simulink model "CheckMate_clipboard"  (R2013a)
settings: Solver=ode23t  StartTime=0.0  StopTime=13.0  RelTol=1e-3
PreLoadFcn:
  | setup_boing
libraries: cmlib x5, simulink x1
Description:
  | CheckMate model of ball bouncing on a surface. Compare this
  | model with the Matalab/Simulink model bounce_smlnk.mdl. See
  | also boing_condition.mdl for an alternative CheckMate
  | model that uses conditions rather than events.
settings Model: Creator=Zhan  LastModifiedBy=zhan
settings DataIOCC: SignalLoggingSaveFormat=ModelDataLogs  SignalLoggingName=sigsOut
settings OptimizationCC: BlockReduction=off  ExpressionDepthLimit=2147483647  InitFltsAndDblsToZero=on
settings DebuggingCC: SaveWithParameterizedLinksMsg=none  SignalResolutionControl=TryResolveAllWithWarning  SolverPrmCheckMsg=none  MultiTaskDSMMsg=warning  MultiTaskCondExecSysMsg=none  FcnCallInpInsideContextMsg=UseLocalSettings  StrictBusMsg=None
settings HardwareCC: TargetUnknown=on
settings SFSimCC: SimParseCustomCode=off
settings RTWCC: IncludeERTFirstTime=on
settings GRTTargetCC: CombineOutputUpdateFcns=off  GRTInterface=on

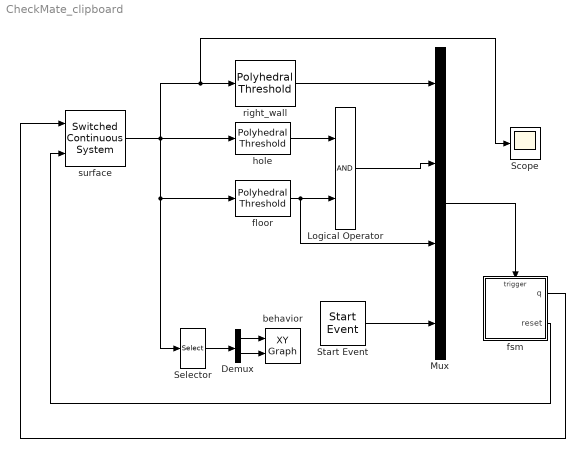
== system CheckMate_clipboard ==
  Demux : Demux  Outputs=2
  Logical Operator : Logic
  Mux : Mux
  Scope : Scope
  Selector : Selector  InputPortWidth=3  IndexOptions=Index vector (dialog)  Indices=[1 2]  OutputSizes=1
  Start Event : cmlib/Start Event  steptime=1  initval=0  finival=1  sampletime=0  interpret=on  enable=on
  behavior : simulink/Sinks/XY Graph  xmin=0  xmax=5  ymin=0  ymax=3  st=-1
  floor : cmlib/Polyhedral Threshold  polyhedron=floor
  fsm : Stateflow chart  TreatAsAtomicUnit=on
  hole : cmlib/Polyhedral Threshold  polyhedron=hole
  right_wall : cmlib/Polyhedral Threshold  polyhedron=right_wall
  surface : cmlib/Switched Continuous System  nx=3  use_sd=off  nup=[]  nz=[]  use_reset=on  nu=1  x0=[0;1+sqrt(2);0]  swfunc=boingfunc  ICS=boing_ICS  AR=boing_AR  use_param=off  p0=[]  PaCs=[]
  wires:
  Mux/1 -> fsm/Trigger
  fsm/2(reset) -> surface/2
  surface/1 -> hole/1, floor/1, Selector/1, right_wall/1, Scope/1
  Start Event/1 -> Mux/4
  fsm/1(q) -> surface/1
  hole/1 -> Logical Operator/1
  floor/1 -> Logical Operator/2, Mux/3
  Logical Operator/1 -> Mux/2
  Selector/1 -> Demux/1
  Demux/1 -> behavior/1
  Demux/2 -> behavior/2
  right_wall/1 -> Mux/1

== stateflow chart CheckMate_clipboard/fsm ==
  state idle1
    entry:q=1;
  state avoid
    entry:q=2;
  state end
    entry:q=3;
  (default) -> idle1 : start
  idle1 -> avoid [order 3] : plop
  idle1 -> end [order 1] : end
  idle1 -> idle1 [order 2] : boing/reset;
  data: q output double
  events: end input RISING_EDGE_EVENT; plop input RISING_EDGE_EVENT; boing input RISING_EDGE_EVENT; start input RISING_EDGE_EVENT; reset output EITHER_EDGE_EVENT
